simulink model "TFlex_ISSGP"  (R2018b)
settings: Solver=VariableStepAuto  StartTime=0.0  StopTime=t_end  RelTol=1e-3
values from neighbouring files (symbols this model uses):
  beta_init = 1    [TFlex_ISSGP_Twin_init.m]    (also in TFlex_ISSGP_init.m)
  beta_min = 0.0000    (= 0)    [TFlex_ISSGP_Twin_init.m]    (also in TFlex_ISSGP_init.m)
  beta_reduc = 0.991    [TFlex_ISSGP_Twin_init.m]    (also in TFlex_ISSGP_init.m = nthroot(beta_T/beta_init,(t_hypUpdate(2)-t_hypUpdate(1))/ts_)
  bufferResamp = 50    [TFlex_ISSGP_Twin_init.m]    (also in TFlex_ISSGP_init.m = 10)
  bufferSize = 25    [TFlex_ISSGP_Twin_init.m]    (also in TFlex_ISSGP_init.m = 250)
  D = 80    [TFlex_ISSGP_Twin_init.m]    (also in TFlex_ISSGP_init.m)
  D_opti = 40    [TFlex_ISSGP_init.m]
  ell = ones(1,n).*0.1    [TFlex_ISSGP_Twin_init.m]    (also in TFlex_ISSGP_init.m = [0.5091   0.0036538   0.0012249])
  ell_init = ell    [TFlex_ISSGP_Twin_init.m]    (also in TFlex_ISSGP_init.m)
  mu_X = [0,0,0]    [TFlex_ISSGP_Twin_init.m]    (also in TFlex_ISSGP_init.m)
  mu_Y = 0    [TFlex_ISSGP_Twin_init.m]    (also in TFlex_ISSGP_init.m)
  n = 3    [TFlex_ISSGP_Twin_init.m]    (also in TFlex_ISSGP_init.m)
  RAND = randn(D,n)    [TFlex_ISSGP_Twin_init.m]    (also in TFlex_ISSGP_init.m)
  RAND_opti = randn(D_opti,n)    [TFlex_ISSGP_init.m]
  sf = 1    [TFlex_ISSGP_Twin_init.m]    (also in TFlex_ISSGP_init.m = 111.9926)
  sf_init = sf    (= 1)    [TFlex_ISSGP_Twin_init.m]    (also in TFlex_ISSGP_init.m = 111.9926)
  sig_X = [1,1,1]    [TFlex_ISSGP_Twin_init.m]    (also in TFlex_ISSGP_init.m)
  sig_Y = 1    [TFlex_ISSGP_Twin_init.m]    (also in TFlex_ISSGP_init.m)
  SIGMA_init = RAND.*ell    [TFlex_ISSGP_Twin_init.m]    (also in TFlex_ISSGP_init.m)
  sn = 2.303584    [TFlex_ISSGP_Twin_init.m]    (also in TFlex_ISSGP_init.m)
  t_hypUpdate = [10 55]    [TFlex_ISSGP_Twin_init.m]    (also in TFlex_ISSGP_init.m = [t_end t_end+1])
  t_learn = 55    [TFlex_ISSGP_Twin_init.m]    (also in TFlex_ISSGP_init.m = 5)
  t_predict = 65    [TFlex_ISSGP_Twin_init.m]    (also in TFlex_ISSGP_init.m = 15)
  ts = 1/1000    (= 0.001)    [TFlex_ISSGP_Twin_init.m]    (also in TFlex_ISSGP_init.m)
  ts_opti = ts*100    (= 0.1)    [TFlex_ISSGP_Twin_init.m]    (also in TFlex_ISSGP_init.m)
  Z = bufferSize*bufferResamp    (= 1250)    [TFlex_ISSGP_Twin_init.m]    (also in TFlex_ISSGP_init.m = 2500)
undefined symbols (not defined in the file or in its folder): Cogging, DiscIntNeverNeededParam, I_limit, PID, Plant, R1, R2, Reference, SVF, X, Y
libraries: simulink x4
settings Model: Creator=wout7  LastModifiedBy=wout7

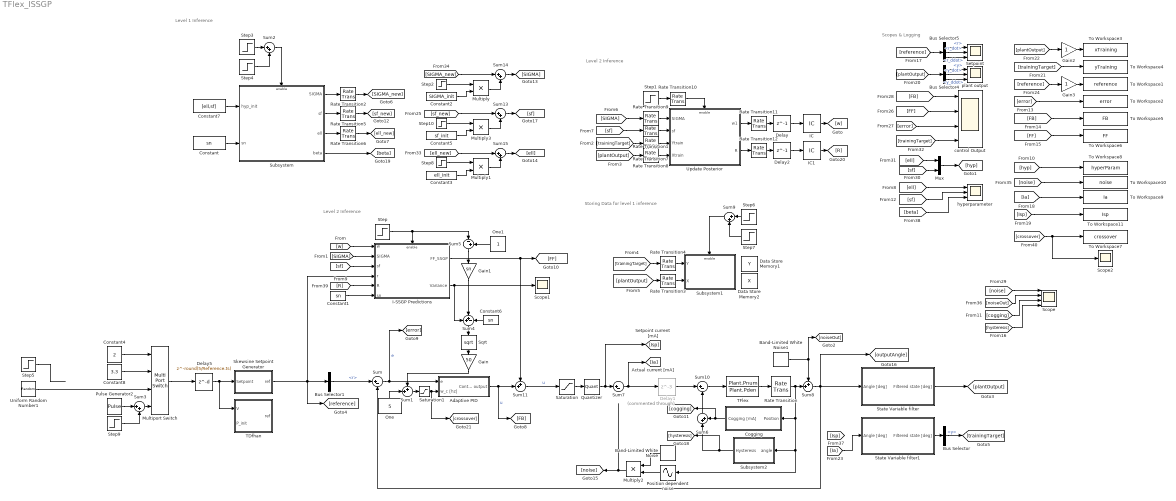
== system TFlex_ISSGP ==
  note: Storing Data for level 1 inference
  note: Scopes & Logging
  note: Level 1 Inference
  note: Level 2 Inference
  note: Level 2 Inference
  Adaptive PID : Subsystem
  Band-Limited White Noise : simulink/Sources/Band-Limited White Noise  Cov=[1e-3]  Ts=ts  seed=48124
  Band-Limited White Noise1 : simulink/Sources/Band-Limited White Noise  Cov=[1e-9]  Ts=ts  seed=[23341]
  Bus Selector : BusSelector  OutputSignals=y
  Bus Selector1 : BusSelector  OutputSignals=r
  Bus Selector4 : BusSelector  OutputSignals=y,y_dot,y_ddot
  Bus Selector5 : BusSelector  OutputSignals=r,r_dot,r_ddot
  Cogging : Subsystem
  Constant : Constant  Value=sn  SampleTime=ts_opti
  Constant1 : Constant  Value=sn  SampleTime=ts_opti
  Constant2 : Constant  Value=SIGMA_init  SampleTime=ts_opti
  Constant3 : Constant  Value=ell_init  SampleTime=ts_opti
  Constant4 : Constant  Value=2  SampleTime=Reference.ts
  Constant5 : Constant  Value=sf_init  SampleTime=ts_opti
  Constant6 : Constant  Value=sn  SampleTime=ts_opti
  Constant7 : Constant  Value=[ell,sf]  VectorParams1D=off  SampleTime=ts_opti
  Constant8 : Constant  Value=3.3  SampleTime=Reference.ts
  Data Store Memory1 : DataStoreMemory  DataStoreName=Y  ReadBeforeWriteMsg=warning  WriteAfterWriteMsg=warning  WriteAfterReadMsg=warning  InitialValue=zeros(bufferSize,1)  VectorParams1D=off  ShowAdditionalParam=off  OutDataTypeStr=double
      settings: LockScale=on
  Data Store Memory2 : DataStoreMemory  DataStoreName=X  ReadBeforeWriteMsg=warning  WriteAfterWriteMsg=warning  WriteAfterReadMsg=warning  InitialValue=zeros(bufferSize,3)  VectorParams1D=off  ShowAdditionalParam=off  OutDataTypeStr=double
      settings: LockScale=on
  Delay : Delay  DelayLength=1  InitialCondition=0
  Delay1 : Delay  Commented=through  DelayLength=3  InitialCondition=0
  Delay2 : Delay  DelayLength=1  InitialCondition=0
  Delay5 : Delay  DelayLength=round(5/Reference.ts)  SampleTime=Reference.ts
  Gain : Gain  Gain=50
  Gain1 : Gain  Gain=sn
  Gain2 : Gain
  Gain3 : Gain
  I-SSGP Predictions : Subsystem
  IC : InitialCondition  Value=ones(2*D,1)*sn
  IC1 : InitialCondition  Value=eye(2*D,2*D).*sn
  Multiply{,1..3} (4 alike) : Product
  Multiport Switch : MultiPortSwitch
  Mux : Mux  Inputs=2
  One : Constant  Value=5  OutDataTypeStr=Inherit: Inherit via back propagation
  One1 : Constant  OutDataTypeStr=Inherit: Inherit via back propagation
  Position dependent noise : Sin  TimeSource=Use external signal  Amplitude=2.5  Bias=7.4979  Frequency=2*pi/13  SampleTime=0
  Pulse Generator2 : DiscretePulseGenerator  Amplitude=2*24  SampleTime=Reference.ts
  Quantizer : Quantizer  QuantizationInterval=1
  Rate Transition{,2,5..6} (4 alike) : RateTransition  OutPortSampleTime=ts
  Rate Transition{1,7..10} (5 alike) : RateTransition  OutPortSampleTime=ts_learn
  Rate Transition11 : RateTransition
  Rate Transition12 : RateTransition
  Rate Transition3 : RateTransition  OutPortSampleTime=ts*bufferResamp
  Rate Transition4 : RateTransition  OutPortSampleTime=ts*bufferResamp
  Saturation : Saturate  UpperLimit=I_limit  LowerLimit=-I_limit
  Saturation1 : Saturate  UpperLimit=35  LowerLimit=0
  Scope : Scope  NumInputPorts=4
  Scope1 : Scope
  Scope2 : Scope
  Setpoint : Scope  NumInputPorts=3
  Skewsine Setpoint Generator : Subsystem
  Sqrt : Sqrt  SaturateOnIntegerOverflow=on
  State Variable filter : Subsystem
  State Variable filter1 : Subsystem
  Step : Step  Time=t_predict  SampleTime=ts
  Step1 : Step  Time=t_learn  SampleTime=ts
  Step10 : Step  Time=t_hypUpdate(1)+ts  Before=1  After=0  SampleTime=ts_opti
  Step2 : Step  Time=t_hypUpdate(1)+ts  Before=1  After=0  SampleTime=ts_opti
  Step3 : Step  Time=t_hypUpdate(2)  After=-1  SampleTime=ts_opti
  Step4 : Step  Time=t_hypUpdate(1)  SampleTime=ts_opti
  Step5 : Step  Time=50  Before=0.5  After=2  SampleTime=0
  Step6 : Step  Time=t_hypUpdate(2)  After=-1  SampleTime=ts_opti
  Step7 : Step  Time=t_hypUpdate(1)-Z*ts  SampleTime=ts_opti
  Step8 : Step  Time=t_hypUpdate(1)+ts  Before=1  After=0  SampleTime=ts_opti
  Step9 : Step  Time=0  After=-24  SampleTime=Reference.ts
  Subsystem : Subsystem
  Subsystem1 : Subsystem
  Subsystem2 : Subsystem
  Sum : Sum  Inputs=|+-
  Sum1 : Sum  Inputs=++|
  Sum10 : Sum  Inputs=|+-
  Sum11 : Sum  Inputs=++|
  Sum{2..3,6,9,13..15} (7 alike) : Sum  Inputs=|++
  Sum4 : Sum  Inputs=++-
  Sum5 : Sum  Inputs=|-+
  Sum7 : Sum  Inputs=|+-
  Sum8 : Sum  Inputs=++|
  TDfhan : Subsystem
  TFlex : TransferFcn  Numerator=Plant.Pnum  Denominator=Plant.Pden  ContinuousStateAttributes='angle'
  To Workspace1 : ToWorkspace  VariableName=reference  SampleTime=-1
  To Workspace10 : ToWorkspace  VariableName=noise  SampleTime=-1
  To Workspace11 : ToWorkspace  VariableName=Isp  SampleTime=-1
  To Workspace2 : ToWorkspace  VariableName=error  SampleTime=-1
  To Workspace3 : ToWorkspace  VariableName=xTraining  SampleTime=-1
  To Workspace4 : ToWorkspace  VariableName=yTraining  SampleTime=-1
  To Workspace5 : ToWorkspace  VariableName=FB  SampleTime=-1
  To Workspace6 : ToWorkspace  VariableName=FF  SampleTime=-1
  To Workspace7 : ToWorkspace  VariableName=crossover  SampleTime=-1
  To Workspace8 : ToWorkspace  VariableName=hyperParam  SampleTime=-1
  To Workspace9 : ToWorkspace  VariableName=Ia  SampleTime=-1
  Uniform Random Number1 : UniformRandomNumber  Minimum=-23  Maximum=23  Seed=Reference.seed  SampleTime=Reference.ts
  Update Posterior : Subsystem
  control Output : Scope  NumInputPorts=4
  hyperparameter : Scope  NumInputPorts=3
  plant output : Scope  NumInputPorts=3
  wires:
  Sum/1 -> Adaptive PID/1(e), [error]  "e"
  Sum8/1 -> State Variable filter/1(Angle [deg]), [outputAngle], Sum/2
  Bus Selector1/1 -> Sum/1  "<r>"
  Step/1 -> Sum5/1, I-SSGP Predictions/Enable
  Step1/1 -> Rate Transition10/1
  IC/1 -> [w]
  [w] -> I-SSGP Predictions/1(w)
  [SIGMA] -> I-SSGP Predictions/2(SIGMA)
  Delay/1 -> IC/1
  [SIGMA] -> Rate Transition9/1
  Constant7/1 -> Subsystem/1(hyp_init)
  Sum2/1 -> Subsystem/Enable
  [sf] -> I-SSGP Predictions/3(sf)
  TFlex/1 -> Rate Transition/1
  [reference] -> Gain3/1
  Bus Selector5/2 -> Setpoint/2  "<r_dot>"
  Bus Selector5/1 -> Setpoint/1  "<r>"
  [error] -> To Workspace2/1
  Bus Selector5/3 -> Setpoint/3  "<r_ddot>"
  [FB] -> To Workspace5/1
  [plantOutput] -> Gain2/1
  Gain2/1 -> To Workspace3/1
  [plantOutput] -> Bus Selector4/1
  Gain3/1 -> To Workspace1/1
  Bus Selector4/1 -> plant output/1  "<y>"
  Bus Selector4/3 -> plant output/3  "<y_ddot>"
  [reference] -> Bus Selector5/1
  [trainingTarget] -> To Workspace4/1
  Bus Selector4/2 -> plant output/2  "<y_dot>"
  [FF] -> To Workspace6/1
  [trainingTarget] -> control Output/4
  [FF] -> control Output/2
  [error] -> control Output/3
  [FB] -> control Output/1
  Step7/1 -> Sum9/2
  Sum9/1 -> Subsystem1/Enable
  Step6/1 -> Sum9/1
  Subsystem/2(sf) -> Rate Transition5/1
  Subsystem/1(SIGMA) -> Rate Transition2/1
  Subsystem/3(ell) -> Rate Transition6/1
  [ell] -> hyperparameter/1
  [hyp] -> To Workspace8/1
  [sf] -> hyperparameter/2
  [sf] -> Mux/2
  [ell] -> Mux/1
  Mux/1 -> [hyp]
  [plantOutput] -> Rate Transition3/1
  Rate Transition3/1 -> Subsystem1/2(X)
  [trainingTarget] -> Rate Transition4/1
  Rate Transition4/1 -> Subsystem1/1(Y)
  Rate Transition2/1 -> [SIGMA_new]
  Rate Transition5/1 -> [sf_new]
  Rate Transition6/1 -> [ell_new]
  [SIGMA_new] -> Sum14/1
  Step2/1 -> Multiply/1
  Constant2/1 -> Multiply/2
  Multiply/1 -> Sum14/2
  Sum14/1 -> [SIGMA]
  Saturation/1 -> Quantizer/1
  Adaptive PID/1(Control output) -> Sum11/2, [FB]  "u"
  State Variable filter/1(Filtered state [deg]) -> [plantOutput]
  Rate Transition/1 -> Sum8/2, Cogging/1(Position), Subsystem2/1(angle), Position dependent noise/1
  Sum11/1 -> Saturation/1  "u"
  Sum10/1 -> TFlex/1
  State Variable filter1/1(Filtered state [deg]) -> Bus Selector/1
  Sum7/1 -> Delay1/1, [Ia]
  Multiply2/1 -> [noise]
  [sf_new] -> Sum13/1
  Step10/1 -> Multiply3/1
  Multiply3/1 -> Sum13/2
  Sum13/1 -> [sf]
  Constant5/1 -> Multiply3/2
  [ell_new] -> Sum15/1
  Step8/1 -> Multiply1/1
  Multiply1/1 -> Sum15/2
  Sum15/1 -> [ell]
  Constant3/1 -> Multiply1/2
  Cogging/1(Cogging [mA]) -> [cogging], Sum6/2
  Quantizer/1 -> [Isp], Sum7/1
  I-SSGP Predictions/1(FF_SSGP) -> Sum11/1, [FF]
  Band-Limited White Noise/1 -> Multiply2/1
  Position dependent noise/1 -> Multiply2/2
  Constant/1 -> Subsystem/2(sn)
  [noise] -> To Workspace10/1
  Pulse Generator2/1 -> Sum3/1
  Sum3/1 -> Multiport Switch/4
  Step9/1 -> Sum3/2
  Constant4/1 -> Multiport Switch/1
  Uniform Random Number1/1 -> Multiport Switch/3
  Constant8/1 -> Multiport Switch/2
  [Ia] -> To Workspace9/1
  [Isp] -> To Workspace11/1
  Band-Limited White Noise1/1 -> [noiseOut], Sum8/1
  Delay1/1 -> Sum10/1
  [Ia] -> State Variable filter1/1(Angle [deg])
  Bus Selector/1 -> [trainingTarget]  "<y>"
  Sum6/1 -> Sum10/2
  [noise] -> Scope/1
  [noiseOut] -> Scope/2
  [cogging] -> Scope/3
  [hysteresis] -> Scope/4
  Subsystem2/1(Hysteresis) -> Sum6/1, [hysteresis]
  Skewsine Setpoint Generator/1(ref) -> [reference], I-SSGP Predictions/4(r), Bus Selector1/1
  Multiport Switch/1 -> Delay5/1
  Delay5/1 -> TDfhan/1(V), Skewsine Setpoint Generator/1(Setpoint)
  [trainingTarget] -> Rate Transition7/1
  [plantOutput] -> Rate Transition8/1
  [sf] -> Rate Transition1/1
  Rate Transition9/1 -> Update Posterior/1(SIGMA)
  Rate Transition10/1 -> Update Posterior/Enable
  Update Posterior/1(w1) -> Rate Transition11/1
  Rate Transition1/1 -> Update Posterior/2(sf)
  Rate Transition7/1 -> Update Posterior/3(Ytrain)
  Rate Transition8/1 -> Update Posterior/4(Xtrain)
  Rate Transition11/1 -> Delay/1
  Step4/1 -> Sum2/2
  Step3/1 -> Sum2/1
  Subsystem/4(beta) -> [beta]
  [beta] -> hyperparameter/3
  Delay2/1 -> IC1/1
  IC1/1 -> [R]
  Rate Transition12/1 -> Delay2/1
  Update Posterior/2(R) -> Rate Transition12/1
  [R] -> I-SSGP Predictions/5(R)
  Constant1/1 -> I-SSGP Predictions/6(sn)
  Step5/1 -> ?
  One/1 -> Sum1/2
  Saturation1/1 -> [crossover], Adaptive PID/2(w_c [hz])
  Sum1/1 -> Saturation1/1
  [crossover] -> Scope2/1, To Workspace7/1
  I-SSGP Predictions/2(Variance) -> Scope1/1, Sum4/1
  Gain/1 -> Sum1/1
  Sqrt/1 -> Gain/1
  Sum4/1 -> Sqrt/1
  One1/1 -> Sum5/2
  Constant6/1 -> Sum4/3
  Sum5/1 -> Gain1/1
  Gain1/1 -> Sum4/2

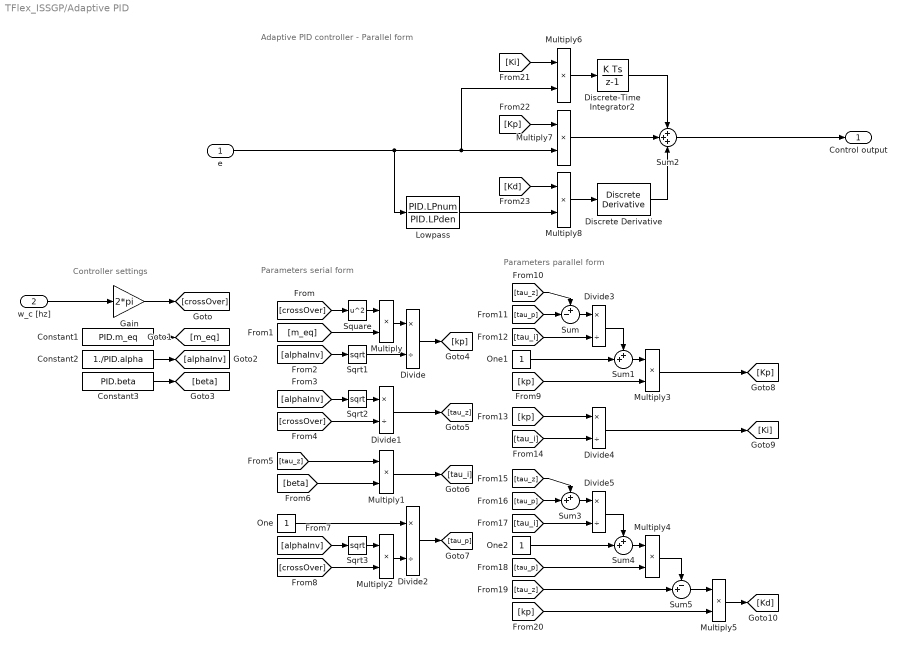
== system TFlex_ISSGP/Adaptive PID ==
  note: Adaptive PID controller - Parallel form
  note: Controller settings
  note: Parameters parallel form
  note: Parameters serial form
  e : Inport
  w_c [hz] : Inport  Port=2
  Constant1 : Constant  Value=PID.m_eq
  Constant2 : Constant  Value=1./PID.alpha
  Constant3 : Constant  Value=PID.beta
  Discrete Derivative : simulink/Discrete/Discrete Derivative  gainval=1.0  ICPrevScaledInput=0.0  OutMin=[]  OutMax=[]  OutDataType=fixdt(1, 16)  OutScaling=2^-10  DoSatur=off
  Discrete-Time Integrator2 : DiscreteIntegrator  SampleTime=-1  ICPrevOutput=DiscIntNeverNeededParam  ICPrevScaledInput=DiscIntNeverNeededParam
  Divide{,1..5} (6 alike) : Product  Inputs=*/
  Gain : Gain  Gain=2*pi
  Lowpass : DiscreteTransferFcn  Numerator=PID.LPnum  Denominator=PID.LPden  SampleTime=ts
  Multiply{,1..8} (9 alike) : Product
  One : Constant  OutDataTypeStr=Inherit: Inherit via back propagation
  One1 : Constant  OutDataTypeStr=Inherit: Inherit via back propagation
  One2 : Constant  OutDataTypeStr=Inherit: Inherit via back propagation
  Sqrt1 : Sqrt  SaturateOnIntegerOverflow=on
  Sqrt2 : Sqrt  SaturateOnIntegerOverflow=on
  Sqrt3 : Sqrt  SaturateOnIntegerOverflow=on
  Square : Math  Operator=square  SaturateOnIntegerOverflow=on
  Sum : Sum  Inputs=+-|
  Sum1 : Sum  Inputs=++|
  Sum2 : Sum  Inputs=3
  Sum3 : Sum  Inputs=++|
  Sum4 : Sum  Inputs=++|
  Sum5 : Sum  Inputs=-+|
  Control output : Outport
  wires:
  w_c [hz]/1 -> Gain/1
  Constant1/1 -> [m_eq]
  Constant2/1 -> [alphaInv]
  Constant3/1 -> [beta]
  [crossOver] -> Square/1
  Square/1 -> Multiply/1
  [m_eq] -> Multiply/2
  [alphaInv] -> Sqrt1/1
  Multiply/1 -> Divide/1
  Sqrt1/1 -> Divide/2
  Divide/1 -> [kp]
  [alphaInv] -> Sqrt2/1
  Sqrt2/1 -> Divide1/1
  [crossOver] -> Divide1/2
  Divide1/1 -> [tau_z]
  [tau_z] -> Multiply1/1
  [beta] -> Multiply1/2
  Multiply1/1 -> [tau_i]
  Sqrt3/1 -> Multiply2/1
  [crossOver] -> Multiply2/2
  [alphaInv] -> Sqrt3/1
  One/1 -> Divide2/1
  Multiply2/1 -> Divide2/2
  Divide2/1 -> [tau_p]
  [tau_z] -> Sum/1
  [tau_p] -> Sum/2
  Sum/1 -> Divide3/1
  [tau_i] -> Divide3/2
  Divide3/1 -> Sum1/1
  One1/1 -> Sum1/2
  Sum1/1 -> Multiply3/1
  [kp] -> Multiply3/2
  Multiply3/1 -> [Kp]
  [kp] -> Divide4/1
  [tau_i] -> Divide4/2
  Divide4/1 -> [Ki]
  [tau_i] -> Divide5/2
  Sum3/1 -> Divide5/1
  [tau_z] -> Sum3/1
  [tau_p] -> Sum3/2
  Divide5/1 -> Sum4/1
  One2/1 -> Sum4/2
  Sum4/1 -> Multiply4/1
  [tau_p] -> Multiply4/2
  Multiply4/1 -> Sum5/1
  [tau_z] -> Sum5/2
  Sum5/1 -> Multiply5/1
  [kp] -> Multiply5/2
  Multiply5/1 -> [Kd]
  Multiply6/1 -> Discrete-Time Integrator2/1
  Sum2/1 -> Control output/1
  e/1 -> Multiply6/2, Multiply7/2, Lowpass/1
  Multiply8/1 -> Discrete Derivative/1
  [Kd] -> Multiply8/1
  Lowpass/1 -> Multiply8/2
  [Kp] -> Multiply7/1
  [Ki] -> Multiply6/1
  Multiply7/1 -> Sum2/2
  Gain/1 -> [crossOver]
  Discrete-Time Integrator2/1 -> Sum2/1
  Discrete Derivative/1 -> Sum2/3

== system TFlex_ISSGP/Cogging ==
  Position : Inport
  Gain : Gain  Gain=20
  Scope : Scope
  Sine Wave Function : Sin  TimeSource=Use external signal  Amplitude=Cogging.amplitude  Frequency=2*pi./Cogging.frequency  Phase=Cogging.phase*2*pi  SampleTime=0
  Sum of Elements : Sum  Inputs=+
  Cogging [mA] : Outport
  wires:
  Gain/1 -> Scope/1, Cogging [mA]/1
  Sum of Elements/1 -> Gain/1
  Position/1 -> Sine Wave Function/1
  Sine Wave Function/1 -> Sum of Elements/1

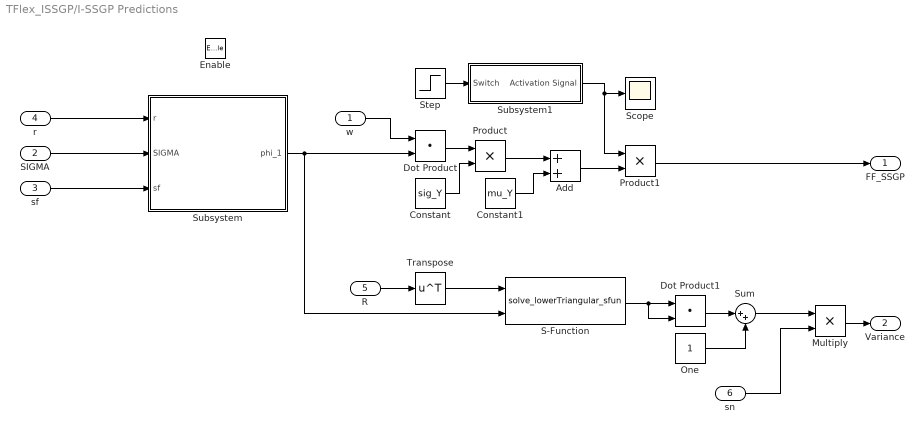
== system TFlex_ISSGP/I-SSGP Predictions ==
  w : Inport
  SIGMA : Inport  Port=2
  sf : Inport  Port=3
  r : Inport  Port=4
  R : Inport  Port=5
  sn : Inport  Port=6
  Enable : EnablePort
  Add : Sum
  Constant : Constant  Value=sig_Y  VectorParams1D=off  SampleTime=ts
  Constant1 : Constant  Value=mu_Y  VectorParams1D=off  SampleTime=ts
  Dot Product : DotProduct  OutDataTypeStr=Inherit: Inherit via internal rule
  Dot Product1 : DotProduct  OutDataTypeStr=Inherit: Inherit via internal rule
  Multiply : Product
  One : Constant  OutDataTypeStr=Inherit: Inherit via back propagation
  Product : Product
  Product1 : Product
  S-Function : S-Function  FunctionName=solve_lowerTriangular_sfun  Parameters=2*D  SFunctionDeploymentMode=off  EnableBusSupport=off
  Scope : Scope
  Step : Step  Time=t_predict  SampleTime=ts
  Subsystem : Subsystem
  Subsystem1 : Subsystem
  Sum : Sum  Inputs=|++
  Transpose : Math  Operator=transpose  SaturateOnIntegerOverflow=on
  FF_SSGP : Outport  SampleTime=ts
  Variance : Outport  Port=2  SampleTime=ts
  wires:
  w/1 -> Dot Product/1
  Subsystem/1(phi_1) -> S-Function/2, Dot Product/2
  SIGMA/1 -> Subsystem/2(SIGMA)
  Dot Product/1 -> Product/1
  Constant/1 -> Product/2
  Product/1 -> Add/1
  Constant1/1 -> Add/2
  Product1/1 -> FF_SSGP/1
  Add/1 -> Product1/2
  sf/1 -> Subsystem/3(sf)
  Subsystem1/1(Activation Signal) -> Product1/1, Scope/1
  r/1 -> Subsystem/1(r)
  Step/1 -> Subsystem1/1(Switch)
  R/1 -> Transpose/1
  Transpose/1 -> S-Function/1
  S-Function/1 -> Dot Product1/1, Dot Product1/2
  sn/1 -> Multiply/2
  Multiply/1 -> Variance/1
  Dot Product1/1 -> Sum/1
  Sum/1 -> Multiply/1
  One/1 -> Sum/2

== system TFlex_ISSGP/Skewsine Setpoint Generator ==
  Setpoint : Inport
  Bus Creator : BusCreator  Inputs=3
  Subsystem : Subsystem
  ref : Outport
  wires:
  Subsystem/3(r_ddot) -> Bus Creator/3  "r_ddot"
  Bus Creator/1 -> ref/1
  Subsystem/2(r_dot) -> Bus Creator/2  "r_dot"
  Subsystem/1(r) -> Bus Creator/1  "r"
  Setpoint/1 -> Subsystem/1(setpoint)

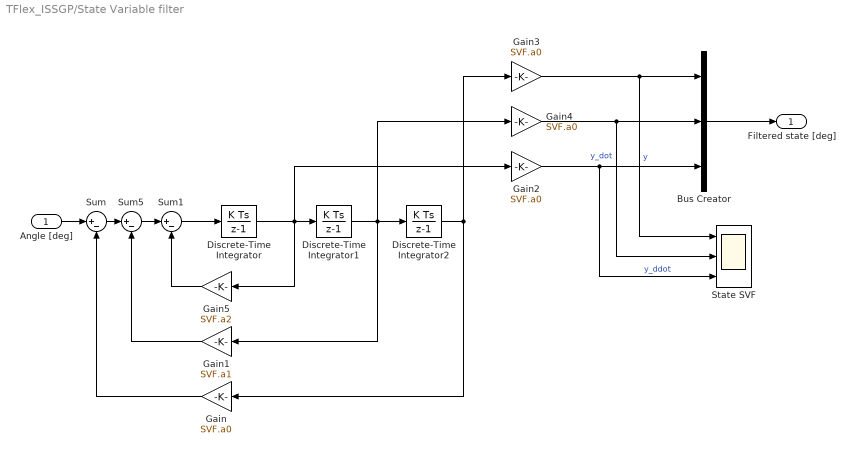
== system TFlex_ISSGP/State Variable filter ==
  Angle [deg] : Inport
  Bus Creator : BusCreator  Inputs=3
  Discrete-Time Integrator : DiscreteIntegrator  SampleTime=-1  ICPrevOutput=DiscIntNeverNeededParam  ICPrevScaledInput=DiscIntNeverNeededParam
  Discrete-Time Integrator1 : DiscreteIntegrator  SampleTime=-1  ICPrevOutput=DiscIntNeverNeededParam  ICPrevScaledInput=DiscIntNeverNeededParam
  Discrete-Time Integrator2 : DiscreteIntegrator  SampleTime=-1  ICPrevOutput=DiscIntNeverNeededParam  ICPrevScaledInput=DiscIntNeverNeededParam
  Gain{,2..4} (4 alike) : Gain  Gain=SVF.a0
  Gain1 : Gain  Gain=SVF.a1
  Gain5 : Gain  Gain=SVF.a2
  State SVF : Scope  NumInputPorts=3
  Sum : Sum  Inputs=|+-
  Sum1 : Sum  Inputs=|+-
  Sum5 : Sum  Inputs=|+-
  Filtered state [deg] : Outport  SampleTime=ts
  wires:
  Bus Creator/1 -> Filtered state [deg]/1
  Sum1/1 -> Discrete-Time Integrator/1
  Angle [deg]/1 -> Sum/1
  Sum/1 -> Sum5/1
  Gain/1 -> Sum/2
  Gain1/1 -> Sum5/2
  Gain3/1 -> State SVF/1, Bus Creator/1  "y"
  Gain2/1 -> State SVF/3, Bus Creator/3  "y_ddot"
  Gain4/1 -> State SVF/2, Bus Creator/2  "y_dot"
  Gain5/1 -> Sum1/2
  Sum5/1 -> Sum1/1
  Discrete-Time Integrator/1 -> Discrete-Time Integrator1/1, Gain2/1, Gain5/1
  Discrete-Time Integrator1/1 -> Discrete-Time Integrator2/1, Gain4/1, Gain1/1
  Discrete-Time Integrator2/1 -> Gain3/1, Gain/1

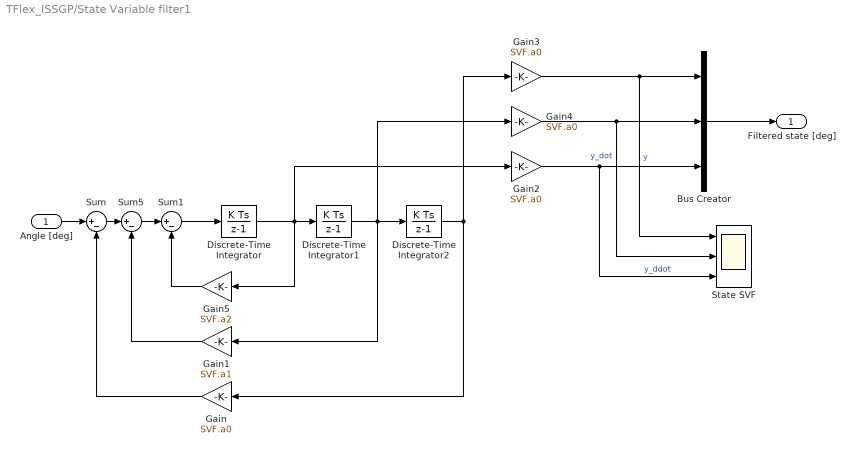
== system TFlex_ISSGP/State Variable filter1 ==
  Angle [deg] : Inport
  Bus Creator : BusCreator  Inputs=3
  Discrete-Time Integrator : DiscreteIntegrator  SampleTime=-1  ICPrevOutput=DiscIntNeverNeededParam  ICPrevScaledInput=DiscIntNeverNeededParam
  Discrete-Time Integrator1 : DiscreteIntegrator  SampleTime=-1  ICPrevOutput=DiscIntNeverNeededParam  ICPrevScaledInput=DiscIntNeverNeededParam
  Discrete-Time Integrator2 : DiscreteIntegrator  SampleTime=-1  ICPrevOutput=DiscIntNeverNeededParam  ICPrevScaledInput=DiscIntNeverNeededParam
  Gain{,2..4} (4 alike) : Gain  Gain=SVF.a0
  Gain1 : Gain  Gain=SVF.a1
  Gain5 : Gain  Gain=SVF.a2
  State SVF : Scope  NumInputPorts=3
  Sum : Sum  Inputs=|+-
  Sum1 : Sum  Inputs=|+-
  Sum5 : Sum  Inputs=|+-
  Filtered state [deg] : Outport  SampleTime=ts
  wires:
  Bus Creator/1 -> Filtered state [deg]/1
  Sum1/1 -> Discrete-Time Integrator/1
  Angle [deg]/1 -> Sum/1
  Sum/1 -> Sum5/1
  Gain/1 -> Sum/2
  Gain1/1 -> Sum5/2
  Gain3/1 -> State SVF/1, Bus Creator/1  "y"
  Gain2/1 -> State SVF/3, Bus Creator/3  "y_ddot"
  Gain4/1 -> State SVF/2, Bus Creator/2  "y_dot"
  Gain5/1 -> Sum1/2
  Sum5/1 -> Sum1/1
  Discrete-Time Integrator/1 -> Discrete-Time Integrator1/1, Gain2/1, Gain5/1
  Discrete-Time Integrator1/1 -> Discrete-Time Integrator2/1, Gain4/1, Gain1/1
  Discrete-Time Integrator2/1 -> Gain3/1, Gain/1

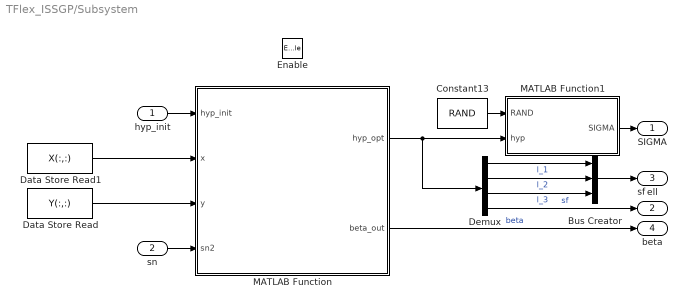
== system TFlex_ISSGP/Subsystem ==
  hyp_init : Inport  PortDimensions=[1,n+1]
  sn : Inport  Port=2
  Enable : EnablePort
  Bus Creator : BusCreator  Inputs=3
  Constant13 : Constant  Value=RAND  VectorParams1D=off  SampleTime=ts_opti
  Data Store Read : DataStoreRead  DataStoreName=Y  SampleTime=ts_opti  DataStoreElements=Y(:,:)
  Data Store Read1 : DataStoreRead  DataStoreName=X  SampleTime=ts_opti  DataStoreElements=X(:,:)
  Demux : Demux
  MATLAB Function : MATLAB Function  TreatAsAtomicUnit=on
  MATLAB Function1 : MATLAB Function  TreatAsAtomicUnit=on
  SIGMA : Outport
  sf : Outport  Port=2
  ell : Outport  Port=3
  beta : Outport  Port=4
  wires:
  hyp_init/1 -> MATLAB Function/1(hyp_init)
  MATLAB Function/2(beta_out) -> beta/1  "beta"
  Data Store Read1/1 -> MATLAB Function/2(x)
  Data Store Read/1 -> MATLAB Function/3(y)
  sn/1 -> MATLAB Function/4(sn2)
  Demux/4 -> sf/1  "sf"
  Constant13/1 -> MATLAB Function1/1(RAND)
  MATLAB Function1/1(SIGMA) -> SIGMA/1
  MATLAB Function/1(hyp_opt) -> Demux/1, MATLAB Function1/2(hyp)
  Demux/1 -> Bus Creator/1  "l_1"
  Demux/2 -> Bus Creator/2  "l_2"
  Demux/3 -> Bus Creator/3  "l_3"
  Bus Creator/1 -> ell/1

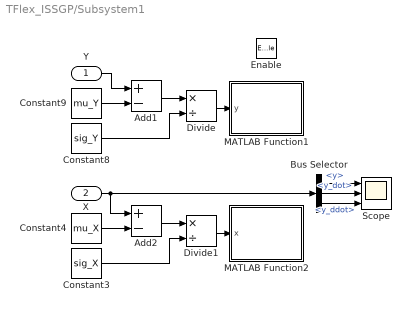
== system TFlex_ISSGP/Subsystem1 ==
  Y : Inport
  X : Inport  Port=2
  Enable : EnablePort
  Add1 : Sum  Inputs=+-
  Add2 : Sum  Inputs=+-
  Bus Selector : BusSelector  OutputSignals=y,y_dot,y_ddot
  Constant3 : Constant  Value=sig_X  VectorParams1D=off  SampleTime=ts_opti
  Constant4 : Constant  Value=mu_X  VectorParams1D=off  SampleTime=ts_opti
  Constant8 : Constant  Value=sig_Y  VectorParams1D=off  SampleTime=ts_opti
  Constant9 : Constant  Value=mu_Y  VectorParams1D=off  SampleTime=ts_opti
  Divide : Product  Inputs=*/
  Divide1 : Product  Inputs=*/
  MATLAB Function1 : MATLAB Function  TreatAsAtomicUnit=on
  MATLAB Function2 : MATLAB Function  TreatAsAtomicUnit=on
  Scope : Scope  NumInputPorts=3
  wires:
  Divide1/1 -> MATLAB Function2/1(x)
  Y/1 -> Add1/1
  Divide/1 -> MATLAB Function1/1(y)
  Add1/1 -> Divide/1
  Add2/1 -> Divide1/1
  Constant9/1 -> Add1/2
  Constant3/1 -> Divide1/2
  Constant4/1 -> Add2/2
  Constant8/1 -> Divide/2
  Bus Selector/1 -> Scope/1  "<y>"
  Bus Selector/2 -> Scope/2  "<y_dot>"
  Bus Selector/3 -> Scope/3  "<y_ddot>"
  X/1 -> Add2/1, Bus Selector/1

== system TFlex_ISSGP/Subsystem2 ==
  angle : Inport
  Discrete Derivative : simulink/Discrete/Discrete Derivative  gainval=1.0  ICPrevScaledInput=0.0  OutMin=[]  OutMax=[]  OutDataType=fixdt(1, 16)  OutScaling=2^-10  DoSatur=off
  Discrete-Time Integrator : DiscreteIntegrator  SampleTime=-1  ICPrevOutput=DiscIntNeverNeededParam  ICPrevScaledInput=DiscIntNeverNeededParam
  MATLAB Function : MATLAB Function  TreatAsAtomicUnit=on
  Sum1 : Sum  Inputs=|+-
  Hysteresis : Outport
  wires:
  MATLAB Function/1(y) -> Sum1/2
  angle/1 -> Discrete Derivative/1
  Sum1/1 -> Discrete-Time Integrator/1
  Discrete Derivative/1 -> Sum1/1, MATLAB Function/1(Vr)
  Discrete-Time Integrator/1 -> Hysteresis/1, MATLAB Function/2(p)

== system TFlex_ISSGP/TDfhan ==
  V : Inport
  P_init : Inport  Port=2
  Bus Creator : BusCreator  Inputs=3
  Constant : Constant  Value=Reference.transient.r  SampleTime=ts
  Constant1 : Constant  Value=Reference.transient.h  SampleTime=ts
  Discrete-Time Integrator : DiscreteIntegrator  gainval=1  SampleTime=ts  ICPrevOutput=DiscIntNeverNeededParam  ICPrevScaledInput=DiscIntNeverNeededParam
  Discrete-Time Integrator1 : DiscreteIntegrator  gainval=1  InitialConditionSource=external  InitialCondition=-24  SampleTime=ts  ICPrevOutput=DiscIntNeverNeededParam  ICPrevScaledInput=DiscIntNeverNeededParam
  MATLAB Function2 : MATLAB Function  TreatAsAtomicUnit=on
  Scope : Scope  NumInputPorts=3
  Sum : Sum  Inputs=+-|
  ref : Outport
  wires:
  Sum/1 -> MATLAB Function2/1(v1)
  V/1 -> Sum/2
  Constant/1 -> MATLAB Function2/3(r0)
  Constant1/1 -> MATLAB Function2/4(h0)
  P_init/1 -> Discrete-Time Integrator1/2
  Discrete-Time Integrator1/1 -> Sum/1, Scope/1, Bus Creator/1  "r"
  Discrete-Time Integrator/1 -> Discrete-Time Integrator1/1, Scope/2, Bus Creator/2, MATLAB Function2/2(v2)  "r_dot"
  Bus Creator/1 -> ref/1
  MATLAB Function2/1(output) -> Scope/3, Bus Creator/3, Discrete-Time Integrator/1  "r_ddot"

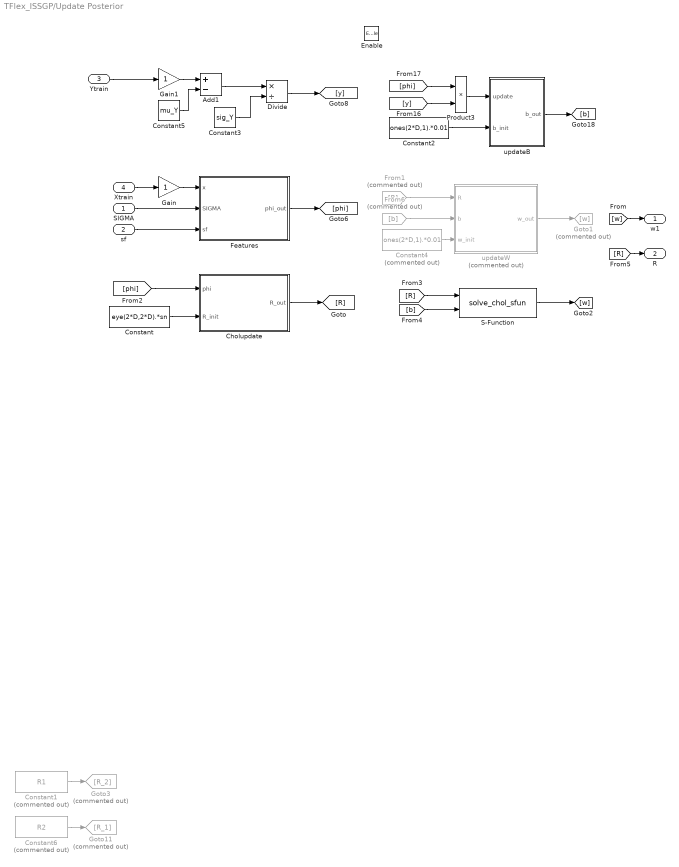
== system TFlex_ISSGP/Update Posterior ==
  SIGMA : Inport
  sf : Inport  Port=2
  Ytrain : Inport  Port=3  PortDimensions=[1,1]
  Xtrain : Inport  Port=4  PortDimensions=[n,1]
  Enable : EnablePort
  Add1 : Sum  Inputs=+-
  Cholupdate : MATLAB Function  TreatAsAtomicUnit=on
  Constant : Constant  Value=eye(2*D,2*D).*sn  SampleTime=-1
  Constant1 : Constant  Commented=on  Value=R1  VectorParams1D=off  SampleTime=-1
  Constant2 : Constant  Value=ones(2*D,1).*0.01  SampleTime=-1
  Constant3 : Constant  Value=sig_Y  VectorParams1D=off  SampleTime=-1
  Constant4 : Constant  Commented=on  Value=ones(2*D,1).*0.01  SampleTime=ts
  Constant5 : Constant  Value=mu_Y  VectorParams1D=off  SampleTime=-1
  Constant6 : Constant  Commented=on  Value=R2  VectorParams1D=off  SampleTime=-1
  Divide : Product  Inputs=*/
  Features : Subsystem
  From1 : From  Commented=on  GotoTag=R
  From6 : From  Commented=on  GotoTag=b
  Gain : Gain
  Gain1 : Gain
  Goto1 : Goto  Commented=on  GotoTag=w
  Goto11 : Goto  Commented=on  GotoTag=R_1
  Goto3 : Goto  Commented=on  GotoTag=R_2
  Product3 : Product
  S-Function : S-Function  FunctionName=solve_chol_sfun  Parameters=2*D  SFunctionDeploymentMode=off  EnableBusSupport=off
  updateB : MATLAB Function  TreatAsAtomicUnit=on
  updateW : MATLAB Function  Commented=on  TreatAsAtomicUnit=on
  w1 : Outport
  R : Outport  Port=2
  wires:
  Divide/1 -> [y]
  [phi] -> Cholupdate/1(phi)
  Features/1(phi_out) -> [phi]
  Cholupdate/1(R_out) -> [R]
  Constant3/1 -> Divide/2
  Constant5/1 -> Add1/2
  Add1/1 -> Divide/1
  From1/1 -> updateW/1(R)
  From6/1 -> updateW/2(b)
  Constant1/1 -> Goto3/1
  Constant6/1 -> Goto11/1
  [y] -> Product3/2
  [phi] -> Product3/1
  Product3/1 -> updateB/1(update)
  updateB/1(b_out) -> [b]
  SIGMA/1 -> Features/2(SIGMA)
  sf/1 -> Features/3(sf)
  Gain/1 -> Features/1(x)
  Gain1/1 -> Add1/1
  Constant/1 -> Cholupdate/2(R_init)
  Constant2/1 -> updateB/2(b_init)
  Constant4/1 -> updateW/3(w_init)
  Ytrain/1 -> Gain1/1
  Xtrain/1 -> Gain/1
  [R] -> S-Function/1
  [b] -> S-Function/2
  [w] -> w1/1
  updateW/1(w_out) -> Goto1/1
  S-Function/1 -> [w]
  [R] -> R/1

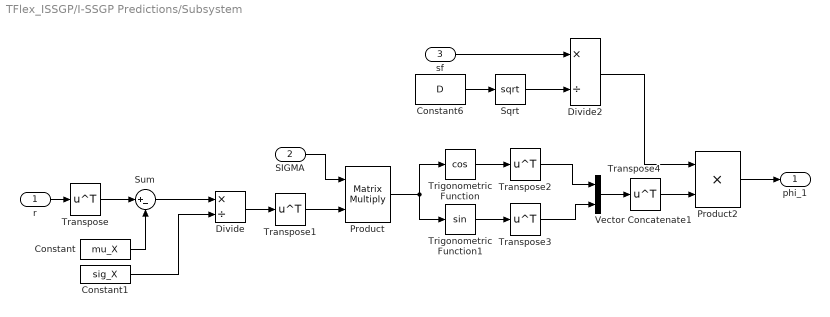
== system TFlex_ISSGP/I-SSGP Predictions/Subsystem ==
  r : Inport
  SIGMA : Inport  Port=2
  sf : Inport  Port=3
  Constant : Constant  Value=mu_X  VectorParams1D=off  SampleTime=-1
  Constant1 : Constant  Value=sig_X  VectorParams1D=off  SampleTime=-1
  Constant6 : Constant  Value=D  SampleTime=-1
  Divide : Product  Inputs=*/
  Divide2 : Product  Inputs=*/
  Product : Product  Multiplication=Matrix(*)
  Product2 : Product
  Sqrt : Sqrt  SaturateOnIntegerOverflow=on
  Sum : Sum  Inputs=|+-
  Transpose{,1..4} (5 alike) : Math  Operator=transpose  SaturateOnIntegerOverflow=on
  Trigonometric Function : Trigonometry  Operator=cos
  Trigonometric Function1 : Trigonometry
  Vector Concatenate1 : Concatenate
  phi_1 : Outport
  wires:
  Transpose1/1 -> Product/2
  Divide/1 -> Transpose1/1
  r/1 -> Transpose/1
  Product/1 -> Trigonometric Function1/1, Trigonometric Function/1
  Product2/1 -> phi_1/1
  sf/1 -> Divide2/1
  Divide2/1 -> Product2/1
  Sum/1 -> Divide/1
  Constant1/1 -> Divide/2
  Constant/1 -> Sum/2
  Transpose2/1 -> Vector Concatenate1/1
  Transpose4/1 -> Product2/2
  Constant6/1 -> Sqrt/1
  Trigonometric Function1/1 -> Transpose3/1
  Trigonometric Function/1 -> Transpose2/1
  Vector Concatenate1/1 -> Transpose4/1
  Transpose3/1 -> Vector Concatenate1/2
  Sqrt/1 -> Divide2/2
  SIGMA/1 -> Product/1
  Transpose/1 -> Sum/1

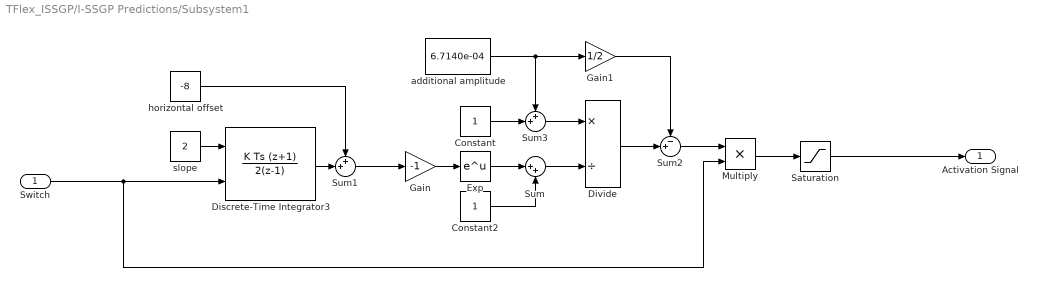
== system TFlex_ISSGP/I-SSGP Predictions/Subsystem1 ==
  Switch : Inport
  Constant : Constant
  Constant2 : Constant
  Discrete-Time Integrator3 : DiscreteIntegrator  IntegratorMethod=Integration: Trapezoidal  ExternalReset=rising  SampleTime=-1  UpperSaturationLimit=1  LowerSaturationLimit=0  ICPrevOutput=DiscIntNeverNeededParam  ICPrevScaledInput=DiscIntNeverNeededParam
  Divide : Product  Inputs=*/
  Exp : Math  SaturateOnIntegerOverflow=on
  Gain : Gain  Gain=-1
  Gain1 : Gain  Gain=1/2
  Multiply : Product
  Saturation : Saturate  UpperLimit=1  LowerLimit=0
  Sum : Sum  Inputs=|++
  Sum1 : Sum  Inputs=++|
  Sum2 : Sum  Inputs=-+|
  Sum3 : Sum  Inputs=++|
  additional amplitude : Constant  Value=6.7140e-04
  horizontal offset : Constant  Value=-8
  slope : Constant  Value=2
  Activation Signal : Outport
  wires:
  Constant/1 -> Sum3/2
  Exp/1 -> Sum/1
  additional amplitude/1 -> Sum3/1, Gain1/1
  Sum1/1 -> Gain/1
  Gain1/1 -> Sum2/1
  Divide/1 -> Sum2/2
  Sum/1 -> Divide/2
  Gain/1 -> Exp/1
  slope/1 -> Discrete-Time Integrator3/1
  Discrete-Time Integrator3/1 -> Sum1/2
  Constant2/1 -> Sum/2
  Sum2/1 -> Multiply/1
  Sum3/1 -> Divide/1
  horizontal offset/1 -> Sum1/1
  Saturation/1 -> Activation Signal/1
  Multiply/1 -> Saturation/1
  Switch/1 -> Multiply/2, Discrete-Time Integrator3/2

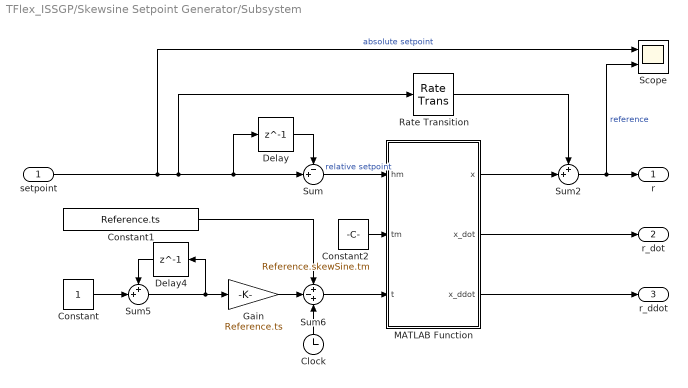
== system TFlex_ISSGP/Skewsine Setpoint Generator/Subsystem ==
  setpoint : Inport
  Clock : Clock
      settings: Decimation=100
  Constant : Constant  SampleTime=Reference.ts
  Constant1 : Constant  Value=Reference.ts  SampleTime=Reference.ts
  Constant2 : Constant  Value=Reference.skewSine.tm  SampleTime=Reference.ts
  Delay : Delay  DelayLength=1  InitialCondition=0  SampleTime=Reference.ts
  Delay4 : Delay  DelayLength=1  InitialCondition=0  SampleTime=Reference.ts
  Gain : Gain  Gain=Reference.ts
  MATLAB Function : MATLAB Function  TreatAsAtomicUnit=on
  Rate Transition : RateTransition  OutPortSampleTime=ts
  Scope : Scope  NumInputPorts=2
  Sum : Sum  Inputs=-+|
  Sum2 : Sum  Inputs=++|
  Sum5 : Sum  Inputs=++|
  Sum6 : Sum  Inputs=+-+
  r : Outport
  r_dot : Outport  Port=2
  r_ddot : Outport  Port=3
  wires:
  Delay4/1 -> Sum5/1
  Sum2/1 -> r/1, Scope/2  "reference"
  Sum5/1 -> Delay4/1, Gain/1
  Constant/1 -> Sum5/2
  MATLAB Function/3(x_ddot) -> r_ddot/1
  Clock/1 -> Sum6/3
  Delay/1 -> Sum/1
  Gain/1 -> Sum6/2
  Constant1/1 -> Sum6/1
  MATLAB Function/2(x_dot) -> r_dot/1
  Sum/1 -> MATLAB Function/1(hm)  "relative setpoint"
  Constant2/1 -> MATLAB Function/2(tm)
  Sum6/1 -> MATLAB Function/3(t)
  MATLAB Function/1(x) -> Sum2/2
  setpoint/1 -> Scope/1, Rate Transition/1, Delay/1, Sum/2  "absolute setpoint"
  Rate Transition/1 -> Sum2/1

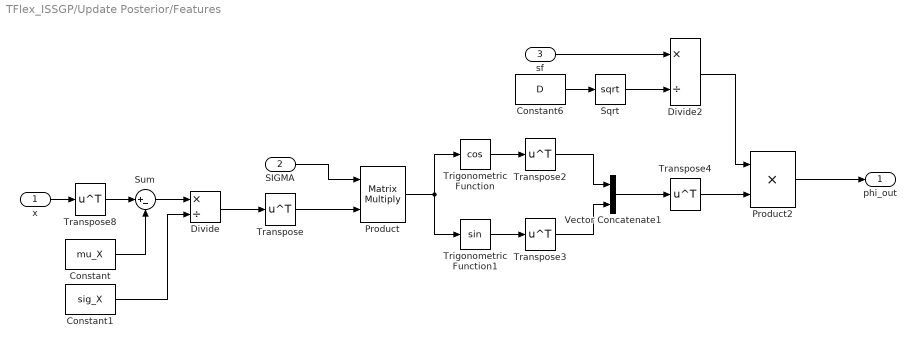
== system TFlex_ISSGP/Update Posterior/Features ==
  x : Inport
  SIGMA : Inport  Port=2
  sf : Inport  Port=3
  Constant : Constant  Value=mu_X  VectorParams1D=off  SampleTime=-1
  Constant1 : Constant  Value=sig_X  VectorParams1D=off  SampleTime=-1
  Constant6 : Constant  Value=D  SampleTime=-1
  Divide : Product  Inputs=*/
  Divide2 : Product  Inputs=*/
  Product : Product  Multiplication=Matrix(*)
  Product2 : Product
  Sqrt : Sqrt  SaturateOnIntegerOverflow=on
  Sum : Sum  Inputs=|+-
  Transpose{,2..4,8} (5 alike) : Math  Operator=transpose  SaturateOnIntegerOverflow=on
  Trigonometric Function : Trigonometry  Operator=cos
  Trigonometric Function1 : Trigonometry
  Vector Concatenate1 : Concatenate
  phi_out : Outport
  wires:
  Sum/1 -> Divide/1
  SIGMA/1 -> Product/1
  Product2/1 -> phi_out/1
  Constant6/1 -> Sqrt/1
  Trigonometric Function1/1 -> Transpose3/1
  Trigonometric Function/1 -> Transpose2/1
  Vector Concatenate1/1 -> Transpose4/1
  Transpose3/1 -> Vector Concatenate1/2
  Product/1 -> Trigonometric Function1/1, Trigonometric Function/1
  Constant1/1 -> Divide/2
  Transpose/1 -> Product/2
  Divide/1 -> Transpose/1
  Divide2/1 -> Product2/1
  Transpose4/1 -> Product2/2
  Sqrt/1 -> Divide2/2
  Constant/1 -> Sum/2
  Transpose2/1 -> Vector Concatenate1/1
  x/1 -> Transpose8/1
  Transpose8/1 -> Sum/1
  sf/1 -> Divide2/1

== matlab function TFlex_ISSGP/Subsystem1/MATLAB Function2 ==
  data: x input; Y data_store_memory; X data_store_memory
function writeTo(x)
global X 

X = [X(2:end,:);x];

== matlab function TFlex_ISSGP/Skewsine Setpoint Generator/Subsystem/MATLAB Function ==
  settings: updateMethod=DISCRETE  sampleTime=ts
  data: hm input; x output; tm input; t input; x_dot output; x_ddot output
function [x,x_dot,x_ddot] = skewSine(hm,tm,t)

if (t>=0) && (t<=tm)
    x      = hm/tm*t - hm/(2*pi)*sin(2*pi/tm*t);
    x_dot  = hm/tm - hm/tm*cos(2*pi/tm*t);
    x_ddot = 2*pi*hm/(tm^2)*sin(2*pi/tm*t);
else
    x      = hm;
    x_dot  = 0;
    x_ddot = 0;
end

== matlab function TFlex_ISSGP/Subsystem/MATLAB Function1 ==
  data: RAND input; SIGMA output; hyp input
function SIGMA  = fcn(RAND,hyp)

SIGMA = zeros(size(RAND));
SIGMA(:,1) = RAND(:,1).*hyp(1);
SIGMA(:,2) = RAND(:,2).*hyp(2);
SIGMA(:,3) = RAND(:,3).*hyp(3);

== matlab function TFlex_ISSGP/Update Posterior/updateW ==
  settings: updateMethod=DISCRETE  sampleTime=ts
  data: R input size=[2*D,2*D]; w_out output size=[2*D,1]; b input; w_init input; D parameter
function w_out = updateW(R,b,w_init,D) 
persistent w
if(isempty(w))
    w = w_init;
end
coder.extrinsic('solve_chol');
w = solve_chol(R,b);
%w = R\(R'\b);
w_out = w;

== matlab function TFlex_ISSGP/Subsystem2/MATLAB Function ==
  data: Vr input; y output; p input
function y = fcn(Vr,p)
if Vr>0 && p>=17
    y = Vr;
elseif Vr<0 && p<=-17
    y = Vr;
else
    y = 0;
end

== matlab function TFlex_ISSGP/Update Posterior/Cholupdate ==
  data: R_out output size=[2*D,2*D]; phi input; R_init input; D parameter; sn parameter
function R_out = cholupdate_fcn(phi, R_init, D, sn)
persistent R; 
if(isempty(R))
    R = R_init;
end
R = cholupdate(R,phi);
R_out = R;

== matlab function TFlex_ISSGP/TDfhan/MATLAB Function2 ==
  data: v1 input; output output; v2 input; r0 input; h0 input
function output = Fhan(v1,v2,r0, h0)
d = h0^2*r0;
a0 = h0*v2;
y = v1 + a0;
a1 = sqrt(d*(d+8*abs(y)));
a2 = a0 + sign(y)*(a1-d)/2;
sy = (sign(y+d)-sign(y-d))/2;
a = (a0+y-a2)*sy +a2;
sa = (sign(a+d)-sign(a-d))/2;
output = -r0 *(a/d -sign(a) )*sa - r0*sign(a);

== matlab function TFlex_ISSGP/Update Posterior/updateB ==
  settings: updateMethod=DISCRETE
  data: update input; b_init input; b_out output size=[2*D,1]; D parameter
function b_out = updateB(update, b_init, D)
persistent b 
if(isempty(b))
    b = b_init;
end

b = b + update;
b_out = b;

== matlab function TFlex_ISSGP/Subsystem/MATLAB Function ==
  data: hyp_init input; hyp_opt output; x input; y input; Z parameter; D_opti parameter; RAND_opti parameter; n parameter; sn2 input; beta_out output; beta_init parameter; beta_min parameter; beta_reduc parameter
function [hyp_opt,beta_out]= hyperparamUpdate(hyp_init,x,y,Z,D_opti,RAND_opti,n,sn2,beta_init, beta_min, beta_reduc)
coder.extrinsic('opt_hyperparam');
persistent hyp1 beta
if(isempty(hyp1))
    hyp1 = hyp_init;
    beta = beta_init;
end
hyp_opt = hyp1;
hyp_new = zeros(size(hyp_init));

hyp_new = opt_hyperparam(hyp_opt,x,y,sn2,Z,D_opti,RAND_opti,n);
hyp1 = hyp_opt.*(1-beta) + beta.*hyp_new;
hyp_opt = hyp1;


beta_new = beta.*beta_reduc;
beta = max(beta_new,beta_min);
beta_out = beta;

== matlab function TFlex_ISSGP/Subsystem1/MATLAB Function1 ==
  data: y input; Y data_store_memory
function writeTo(y)
global Y 

Y = [Y(2:end,:);y'];
